simulink model "Ex3_Function_Compute_Simple"  (R2017a)
settings: Solver=FixedStepAuto  StartTime=-3*pi  StopTime=3*pi  FixedStep=pi/3000  RelTol=1e-3
settings Model: Creator=sulaymon.eshkabilov  LastModifiedBy=sulaymon.eshkabilov

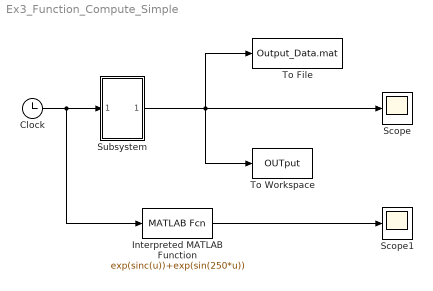
== system Ex3_Function_Compute_Simple ==
  Clock : Clock
  Interpreted MATLAB Function : MATLABFcn  MATLABFcn=exp(sinc(u))+exp(sin(250*u))
  Scope : Scope
  Scope1 : Scope
  Subsystem : Subsystem
  To File : ToFile  Filename=Output_Data.mat  SaveFormat=Timeseries
  To Workspace : ToWorkspace  VariableName=OUTput  SaveFormat=Timeseries  SampleTime=-1
  wires:
  Subsystem/1(Out1) -> Scope/1, To File/1, To Workspace/1
  Clock/1 -> Interpreted MATLAB Function/1, Subsystem/1(In1)
  Interpreted MATLAB Function/1 -> Scope1/1

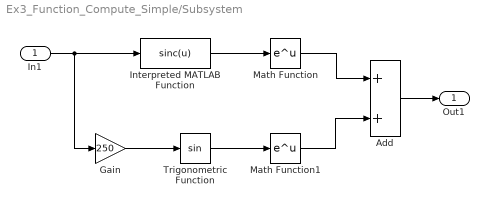
== system Ex3_Function_Compute_Simple/Subsystem ==
  In1 : Inport
  Add : Sum
  Gain : Gain  Gain=250
  Interpreted MATLAB Function : MATLABFcn  MATLABFcn=sinc(u)
  Math Function : Math  SaturateOnIntegerOverflow=on
  Math Function1 : Math  SaturateOnIntegerOverflow=on
  Trigonometric Function : Trigonometry
  Out1 : Outport
  wires:
  Trigonometric Function/1 -> Math Function1/1
  Math Function/1 -> Add/1
  Math Function1/1 -> Add/2
  Add/1 -> Out1/1
  Gain/1 -> Trigonometric Function/1
  In1/1 -> Interpreted MATLAB Function/1, Gain/1
  Interpreted MATLAB Function/1 -> Math Function/1
